simulink model "ex3S"  (R2021b)
settings: Solver=ode45  StartTime=0.0  StopTime=0.5  MaxStep=0.5*10^-2  RelTol=1e-9
values from neighbouring files (symbols this model uses):
  C = 0.0157    [ex2_1.m]    (also in ex3.m = 3.73e-06; ex4.m = [1 0]; mp62.m = [1 0]; od.m = [1 0;0 0])
  c = 0.1    [ex1.m]    (also in ex2_1.m; ex3.m; ex4.m; od.m)
  k = linspace(-5,5,1000)    [OP2_dynamicEstimation.m]    (also in dynamicEstimation.m = x2; ex1.m = 100; ex2_1.m = 100; ex3.m = 1272.8)
  Kd = 0.1    [ex1.m]    (also in ex3.m = 0)
  Kp = 300    [ex1.m]    (also in ex3.m = 1)
  l = dynamicEstimation(x1,y1,x2,y2,10)    [OP2_dynamicEstimation.m]    (also in ex1.m = 0.0003; ex2_1.m = 0.0003; ex3.m = 0.0003)
  m = 1    [ex1.m]    (also in ex2_1.m; ex3.m = 0.48; ex4.m = 0.48; od.m = 0.48)
libraries: slpidlib x1
settings Model: Creator=danli  LastModifiedBy=danli
settings SolverCC: AlgebraicLoopSolver=TrustRegion
settings DebuggingCC: SFMachineParentedDataDiag=warning

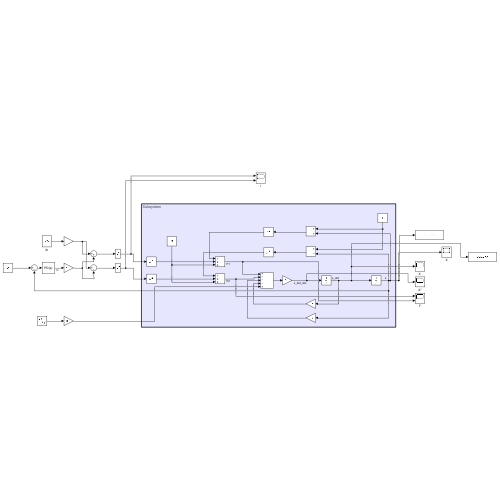
[thumbnail: Simulink's stored preview of the top-level diagram]
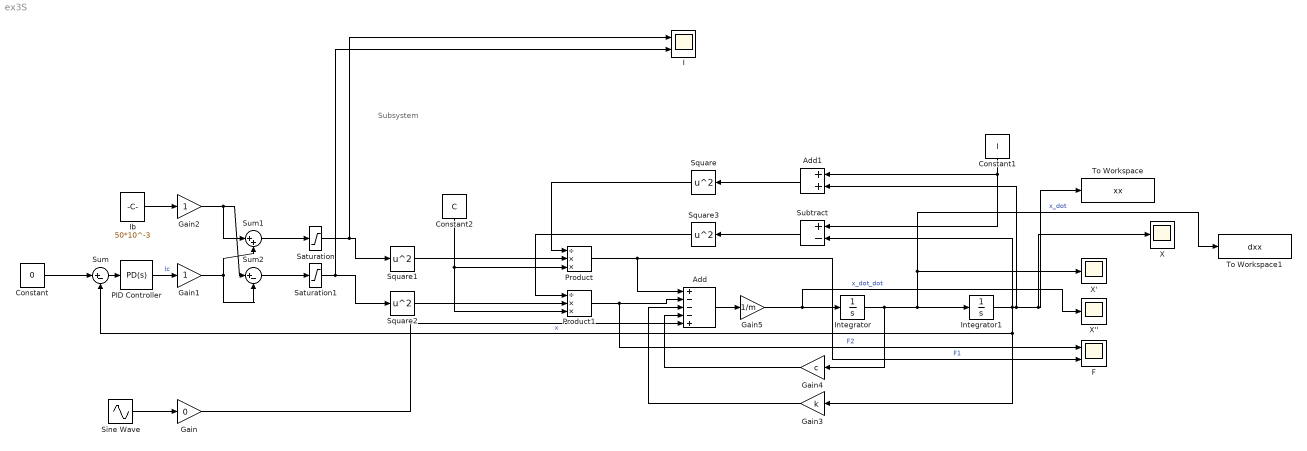
== system ex3S ==
  note: Subsystem
  Add : Sum  Inputs=+---+
  Add1 : Sum
  Constant : Constant  Value=0
  Constant1 : Constant  Value=l
  Constant2 : Constant  Value=C
  F : Scope  NumInputPorts=2
  Gain : Gain  Gain=0
  Gain1 : Gain
  Gain2 : Gain
  Gain3 : Gain  Gain=k
  Gain4 : Gain  Gain=c
  Gain5 : Gain  Gain=1/m
  I : Scope  NumInputPorts=2
  Ib : Constant  Value=50*10^-3
  Integrator : Integrator
  Integrator1 : Integrator  InitialCondition=50*10^-6
  PID Controller : slpidlib/PID Controller  Controller=PD  Form=Parallel  TimeDomain=Continuous-time  UseExternalTs=off  SampleTime=-1  IntegratorMethod=Forward Euler  FilterMethod=Forward Euler  ControllerParametersSource=internal  P=Kp  I=2500  D=Kd  UseFilter=on  N=350  TunerSelectOption=Frequency Response Based  InitialConditionSource=internal  InitialConditionForIntegrator=0  InitialConditionForFilter=0  DifferentiatorICPrevScaledInput=0  ExternalReset=none  TrackingMode=off  Kt=1  LimitOutput=off  SatLimitsSource=internal  UpperSaturationLimit=inf  LowerSaturationLimit=-inf  LinearizeAsGain=on  AntiWindupMode=none  Kb=1  POutMin=[]  POutMax=[]  IOutMin=[]  IOutMax=[]  DOutMin=[]  DOutMax=[]  NOutMin=[]  NOutMax=[]  SumOutMin=[]  SumOutMax=[]  SaturationOutMin=[]  SaturationOutMax=[]  PParamMin=[]  PParamMax=[]  IParamMin=[]  IParamMax=[]  DParamMin=[]  DParamMax=[]  NParamMin=[]  NParamMax=[]  KbParamMin=[]  KbParamMax=[]  KtParamMin=[]  KtParamMax=[]  KbOutMin=[]  KbOutMax=[]  KtOutMin=[]  KtOutMax=[]  IntegratorOutMin=[]  IntegratorOutMax=[]  FilterOutMin=[]  FilterOutMax=[]  SumI1OutMin=[]  SumI1OutMax=[]  SumI2OutMin=[]  SumI2OutMax=[]  SumI3OutMin=[]  SumI3OutMax=[]  SumI4OutMin=[]  SumI4OutMax=[]  SumDOutMin=[]  SumDOutMax=[]  DifferentiatorOutMin=[]  DifferentiatorOutMax=[]  FilterDiffOutCoefMin=[]  FilterDiffOutCoefMax=[]  ReciprocalOutMin=[]  ReciprocalOutMax=[]  SumDenOutMin=[]  SumDenOutMax=[]  SumNumOutMin=[]  SumNumOutMax=[]  DivideOutMin=[]  DivideOutMax=[]  UdiffTsProdOutMin=[]  UdiffTsProdOutMax=[]  NTsProdOutMin=[]  NTsProdOutMax=[]  UintegralTsProdOutMin=[]  UintegralTsProdOutMax=[]  UngainTsProdOutMin=[]  UngainTsProdOutMax=[]  IntegratorContinuousStateAttributes=''  IntegratorStateMustResolveToSignalObject=off  IntegratorRTWStateStorageClass=Auto  FilterContinuousStateAttributes=''  FilterStateMustResolveToSignalObject=off  FilterRTWStateStorageClass=Auto  ParallelPVariant=InternalParameters  IdealPVariant=Disabled  IVariant=Disabled  DVariant=InternalParameters  IntegratorVariant=Disabled  SatVariant=Disabled  AWVariant=Disabled  PCopyVariant=Disabled  TRVariant=Disabled  FdbkBlocksVariant=Forward  IdealPFdbkVariant=Disabled  SatFdbkVariant=Disabled  DerivativeFilterVariant=ContFilter  NVariant=InternalParameters  NCopyVariant=Disabled  FilterICVariant=InternalICsFilter  IntegratorICVariant=Disabled  ExternalResetVariant=Disabled  TRSumVariant=Passthrough  SumFdbkVariant=Disabled  SumVariant=Sum_PD  TsampFilterVariant=InternalTs  TsampNgainVariant=Passthrough  TsampIntegralVariant=Disabled_SignalSpec  ExternalSaturationOutDataTypeStr=Inherit: Same as second input
  Product : Product  Inputs=/**
  Product1 : Product  Inputs=/**
  Saturation : Saturate  UpperLimit=2  LowerLimit=0
  Saturation1 : Saturate  UpperLimit=2  LowerLimit=0
  Sine Wave : Sin  Amplitude=13  Frequency=230  SampleTime=0
  Square{,1..3} (4 alike) : Math  Operator=square  SaturateOnIntegerOverflow=on
  Subtract : Sum  Inputs=+-
  Sum : Sum  Inputs=|+-
  Sum1 : Sum  Inputs=|++
  Sum2 : Sum  Inputs=|+-
  To Workspace : ToWorkspace  VariableName=xx  SaveFormat=Timeseries  SampleTime=-1
  To Workspace1 : ToWorkspace  VariableName=dxx  SaveFormat=Timeseries  SampleTime=-1
  X : Scope
  X' : Scope
  X'' : Scope
  wires:
  Constant/1 -> Sum/1
  Sum/1 -> PID Controller/1
  Sine Wave/1 -> Gain/1
  Ib/1 -> Gain2/1
  Sum1/1 -> Saturation/1
  Sum2/1 -> Saturation1/1
  PID Controller/1 -> Gain1/1  "Ic"
  Gain1/1 -> Sum1/2, Sum2/2
  Gain2/1 -> Sum2/1, Sum1/1
  Gain/1 -> Add/5
  Saturation1/1 -> Square2/1, I/2
  Saturation/1 -> Square1/1, I/1
  Integrator1/1 -> Sum/2, Gain3/1, To Workspace/1, X/1, Add1/2, Subtract/2  "x"
  Square2/1 -> Product1/2
  Constant1/1 -> Subtract/1, Add1/1
  Square1/1 -> Product/2
  Gain4/1 -> Add/4
  Integrator/1 -> X'/1, To Workspace1/1, Integrator1/1, Gain4/1  "x_dot"
  Gain3/1 -> Add/3
  Product1/1 -> F/1, Add/2  "F2"
  Subtract/1 -> Square3/1
  Square/1 -> Product/1
  Add1/1 -> Square/1
  Add/1 -> Gain5/1
  Product/1 -> F/2, Add/1  "F1"
  Square3/1 -> Product1/1
  Constant2/1 -> Product/3, Product1/3
  Gain5/1 -> X''/1, Integrator/1  "x_dot_dot"
